simulink model "TriggerFun1_2018a"  (R2018a)
settings: Solver=VariableStepAuto  StartTime=0.0  StopTime=2.0  RelTol=1e-3
settings Model: Creator=86188  LastModifiedBy=bzhan

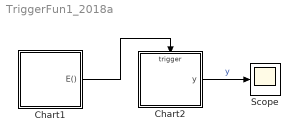
== system TriggerFun1_2018a ==
  Chart1 : Stateflow chart  TreatAsAtomicUnit=on
  Chart2 : Stateflow chart  TreatAsAtomicUnit=on
  Scope : Scope
  wires:
  Chart1/1(E()) -> Chart2/Trigger
  Chart2/1(y) -> Scope/1  "y"

== stateflow chart TriggerFun1_2018a/Chart2 ==
  settings: executeAtInitialization=1
  state A
    en:y = 0;
    du:y = y + 1;
  (default) -> A
  data: y output double =0
  events: E input FUNCTION_CALL_EVENT

== stateflow chart TriggerFun1_2018a/Chart1 ==
  settings: updateMethod=DISCRETE  sampleTime=0.1
  state A
    en:
    f("en_chart1");
    du:f("du_chart1");
    send(E);
  state B
    en:f("en_B");
    du:f("du_B");
  (default) -> A
  A -> B : after(5,tick)
  B -> A : after(5,tick)
  data: s function_input
  events: E output FUNCTION_CALL_EVENT
  function f(s):
    | function f(s)
    |   fprintf(s+"\n");
